simulink library "filteredPIDControllerRes_ul"  (R2020a)
settings: Solver=VariableStepAuto  StartTime=0.0  StopTime=10.0  RelTol=1e-3
undefined symbols (not defined in the file or in its folder): kd, ki, kp, lowerLimit, tau, upperLimit
settings Model: Creator=mcobb  LastModifiedBy=andre
settings DataIOCC: ReturnWorkspaceOutputs=off
settings DebuggingCC: ArithmeticOperatorsInVariantConditions=warning
settings SFSimCC: CustomCodeUndefinedFunction=UseInterfaceOnly

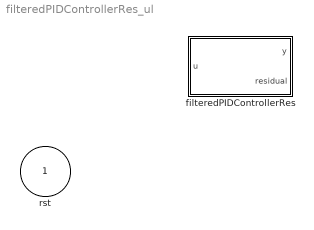
== system filteredPIDControllerRes_ul ==
  rst : Inport
  filteredPIDControllerRes : Subsystem  mask{kp=kp, ki=ki, kd=kd, Value=tau, externalReset=none, UpperLimit=upperLimit, LowerLimit=lowerLimit}
      mask prompts: kp "Proportional Gain, kp"; ki "Integral Gain, ki"; kd "Derivative Gain, kd"; Value "Time Constant, s"; externalReset "External reset:"; UpperLimit "Simulink:blkprm_prompts:SaturateUpLim"; LowerLimit "Simulink:blkprm_prompts:SaturateLowLim"
      mask init:
      | initfcn
      mask TypeOptions kp: kp/Gain
      mask TypeOptions ki: ki/Gain
      mask TypeOptions kd: kd/Gain
      mask TypeOptions Value: tau/Value
      mask TypeOptions externalReset: none | rising | falling | either | level | level hold
      mask TypeOptions UpperLimit: Saturation/UpperLimit
      mask TypeOptions LowerLimit: Saturation/LowerLimit
      mask DialogControl UpperLimit Prompt: Upper limit:
      mask DialogControl LowerLimit Prompt: Lower limit:

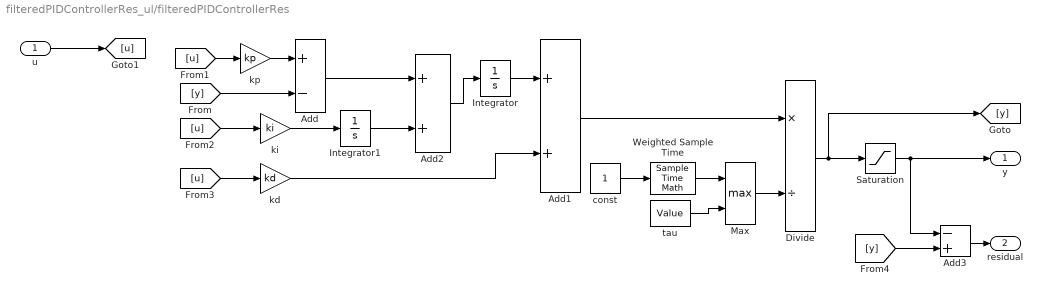
== system filteredPIDControllerRes_ul/filteredPIDControllerRes ==
  u : Inport  PortDimensions=1
  Add : Sum  Inputs=+-
  Add1 : Sum
  Add2 : Sum
  Add3 : Sum  Inputs=-+
  Divide : Product  Inputs=*/
  Integrator : Integrator
  Integrator1 : Integrator
  Max : MinMax  Function=max  Inputs=2
  Saturation : Saturate  UpperLimit=UpperLimit  LowerLimit=LowerLimit
  Weighted Sample Time : SampleTimeMath  TsampMathOp=Ts Only
  const : Constant
  kd : Gain  Gain=kd
  ki : Gain  Gain=ki
  kp : Gain  Gain=kp
  tau : Constant  Value=Value
  y : Outport  PortDimensions=1  VectorParamsAs1DForOutWhenUnconnected=off
  residual : Outport  Port=2
  wires:
  u/1 -> [u]
  kp/1 -> Add/1
  [y] -> Add/2
  [u] -> kp/1
  Max/1 -> Divide/2
  tau/1 -> Max/2
  Integrator1/1 -> Add2/2
  ki/1 -> Integrator1/1
  [u] -> ki/1
  [u] -> kd/1
  kd/1 -> Add1/2
  Add1/1 -> Divide/1
  Divide/1 -> Saturation/1, [y]
  Weighted Sample Time/1 -> Max/1
  const/1 -> Weighted Sample Time/1
  Integrator/1 -> Add1/1
  Add2/1 -> Integrator/1
  Add/1 -> Add2/1
  Saturation/1 -> Add3/1, y/1
  [y] -> Add3/2
  Add3/1 -> residual/1
